simulink model "closed_circuit_simulink"  (R2025b)
settings: Solver=FixedStepDiscrete  StartTime=0.0  StopTime=5  FixedStep=0.01  RelTol=1e-3
values from neighbouring files (symbols this model uses):
  PSD_fresh = PSD_fresh / sum(PSD_fresh)    [Initialisation_simulink.m]    (also in closed_circuit_mill_cyclone.m = data.PSD_fresh_percent(:)' / sum(data.PSD_fresh_percent); closed_circuit_with_pulp.m = PSD_fresh/sum(PSD_fresh))
settings Model: Creator=fabri  LastModifiedBy=fabri
settings DebuggingCC: AlgebraicLoopMsg=none

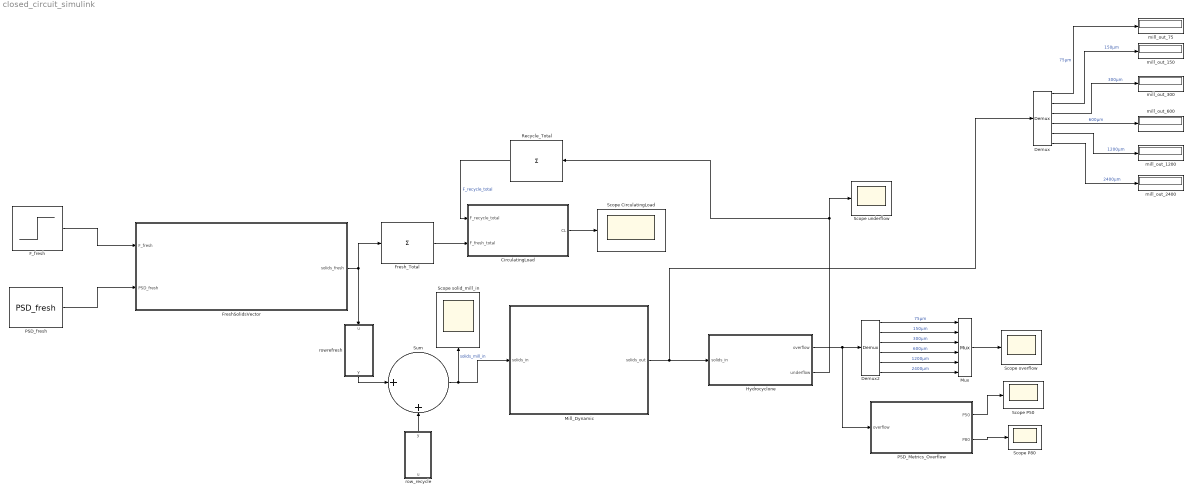
== system closed_circuit_simulink ==
  CirculatingLoad : MATLAB Function  TreatAsAtomicUnit=on
  Demux : Demux  Outputs=6
  Demux2 : Demux  Outputs=6
  F_fresh : Step  Time=2  Before=100  After=120  SampleTime=0
  FreshSolidsVector : MATLAB Function  TreatAsAtomicUnit=on
  Fresh_Total : Sum  Inputs=+
  Hydrocyclone : Subsystem
  Mill_Dynamic : Subsystem
  Mux : Mux  Inputs=6
  PSD_Metrics_Overflow : MATLAB Function  TreatAsAtomicUnit=on
  PSD_fresh : Constant  Value=PSD_fresh
  Recycle_Total : Sum  Inputs=+
  Scope CirculatingLoad : Scope
      settings: ActiveDisplayYMinimum=-0.12499989982802118  ActiveDisplayYMaximum=1.1249990984521909  DataLoggingVariableName=ScopeData3
  Scope P50 : Scope
      settings: ActiveDisplayYMinimum=129.16776995658694  ActiveDisplayYMaximum=136.03382464797281  YLabel=Flow rate (t/h)  DataLoggingVariableName=ScopeData4
  Scope P80 : Scope
      settings: ActiveDisplayYMinimum=262.78762207985039  ActiveDisplayYMaximum=284.16808065274466  YLabel=Flow rate (t/h)  DataLoggingVariableName=ScopeData5
  Scope overflow : Scope
      settings: ActiveDisplayYMinimum=-371.98238867119983  ActiveDisplayYMaximum=1586.5773709597061  YLabel=Flow rate (t/h)
  Scope solid_mill_in : Scope
      settings: ActiveDisplayYMinimum=3.0098879063285189  ActiveDisplayYMaximum=36.512278921953538
  Scope underflow : Scope
      settings: ActiveDisplayYMinimum=-0.69801762722274052  ActiveDisplayYMaximum=1.5006822165423852  DataLoggingVariableName=ScopeData2
  Sum : Sum  Inputs=|++
  mill_out_{75,150,300,600,1200,2400} (6 alike) : Display
  row_recycle : MATLAB Function  TreatAsAtomicUnit=on
  rowrefresh : MATLAB Function  TreatAsAtomicUnit=on
  wires:
  F_fresh/1 -> FreshSolidsVector/1(F_fresh)
  PSD_fresh/1 -> FreshSolidsVector/2(PSD_fresh)
  FreshSolidsVector/1(solids_fresh) -> rowrefresh/1(u), Fresh_Total/1
  Sum/1 -> Mill_Dynamic/1(solids_in), Scope solid_mill_in/1  "solids_mill_in"
  Demux/6 -> mill_out_2400/1  "2400µm"
  Demux/4 -> mill_out_600/1  "600µm"
  Demux/3 -> mill_out_300/1  "300µm"
  Demux/2 -> mill_out_150/1  "150µm"
  Demux/1 -> mill_out_75/1  "75µm"
  Mill_Dynamic/1(solids_out) -> Demux/1, Hydrocyclone/1(solids_in)
  Demux/5 -> mill_out_1200/1  "1200µm"
  Hydrocyclone/2(underflow) -> Scope underflow/1, Recycle_Total/1
  row_recycle/1(y) -> Sum/2
  rowrefresh/1(y) -> Sum/1
  Hydrocyclone/1(overflow) -> Demux2/1, PSD_Metrics_Overflow/1(overflow)
  Demux2/3 -> Mux/3  "300µm"
  Fresh_Total/1 -> CirculatingLoad/2(F_fresh_total)
  Recycle_Total/1 -> CirculatingLoad/1(F_recycle_total)  "F_recycle_total"
  CirculatingLoad/1(CL) -> Scope CirculatingLoad/1
  Mux/1 -> Scope overflow/1
  Demux2/1 -> Mux/1  "75µm"
  Demux2/4 -> Mux/4  "600µm"
  Demux2/2 -> Mux/2  "150µm"
  Demux2/5 -> Mux/5  "1200µm"
  Demux2/6 -> Mux/6  "2400µm"
  PSD_Metrics_Overflow/2(P80) -> Scope P80/1
  PSD_Metrics_Overflow/1(P50) -> Scope P50/1

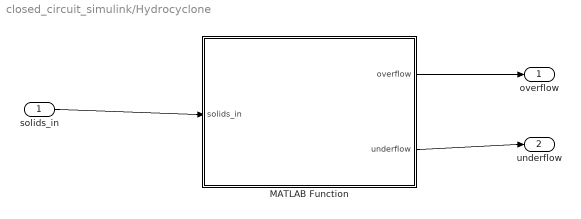
== system closed_circuit_simulink/Hydrocyclone ==
  solids_in : Inport
  MATLAB Function : MATLAB Function  TreatAsAtomicUnit=on
  overflow : Outport
  underflow : Outport  Port=2
  wires:
  solids_in/1 -> MATLAB Function/1(solids_in)
  MATLAB Function/2(underflow) -> underflow/1
  MATLAB Function/1(overflow) -> overflow/1

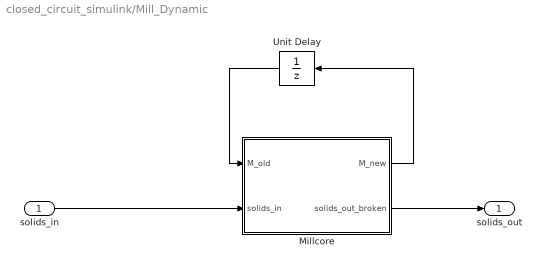
== system closed_circuit_simulink/Mill_Dynamic ==
  solids_in : Inport
  Millcore : MATLAB Function  TreatAsAtomicUnit=on
  Unit Delay : UnitDelay  InitialCondition=[0 0 0 0 0 0]  SampleTime=-1  HasFrameUpgradeWarning=on
  solids_out : Outport
  wires:
  solids_in/1 -> Millcore/2(solids_in)
  Millcore/1(M_new) -> Unit Delay/1
  Millcore/2(solids_out_broken) -> solids_out/1
  Unit Delay/1 -> Millcore/1(M_old)

== matlab function closed_circuit_simulink/Mill_Dynamic/Millcore ==
  data: M_old input; M_new output; solids_in input; solids_out_broken output
function [M_new, solids_out_broken] = MillCore(M_old, solids_in)

% Paramètres
tau = 0.25;
dt  = 0.01;

selection = [0 0.05 0.10 0.20 0.35 0.50];

B = [1   1   0.3 0.1 0   0;
     0   0   0.7 0.3 0.2 0;
     0   0   0   0.6 0.3 0.2;
     0   0   0   0   0.5 0.3;
     0   0   0   0   0   0.5;
     0   0   0   0   0   0];

% Forcer vecteurs ligne
M_old = reshape(M_old, 1, []);
solids_in = reshape(solids_in, 1, []);

% Débit de sortie brut
solids_out_raw = M_old / tau;
F_out = sum(solids_out_raw);

% PSD brute
if F_out > 0
    PSD_raw = solids_out_raw / F_out;
else
    PSD_raw = zeros(size(solids_out_raw));
end

% Application de la cassure
PSD_broken = run_breakage(PSD_raw, selection, B);

% Débit solide broyé en sortie
solids_out_broken = F_out * PSD_broken;

% Bilan dynamique
dMdt = solids_in - solids_out_broken;
M_new = M_old + dt * dMdt;

M_new(M_new < 0) = 0;

end

function PSD_out = run_breakage(PSD_in, selection, B)

n = length(PSD_in);
PSD_out = zeros(1,n);

for j = 1:n
    f = PSD_in(j);
    s = selection(j);

    unbroken = (1-s) * f;
    broken = s * f;

    PSD_out(j) = PSD_out(j) + unbroken;
    PSD_out = PSD_out + broken * B(:,j)';
end

if sum(PSD_out) > 0
    PSD_out = PSD_out / sum(PSD_out);
end

end

== matlab function closed_circuit_simulink/FreshSolidsVector ==
  data: F_fresh input; solids_fresh output; PSD_fresh input
function solids_fresh = FreshSolidsVector(F_fresh, PSD_fresh)

PSD_fresh = reshape(PSD_fresh, 1, []);
solids_fresh = F_fresh .* PSD_fresh;

end

== matlab function closed_circuit_simulink/Hydrocyclone/MATLAB Function ==
  data: solids_in input; overflow output; underflow output
function [overflow, underflow] = CycloneCore(solids_in)

% Paramètre
d50 = 300; % micron (taille de coupure)

size_classes = [75 150 300 600 1200 2400];

% Forcer vecteur ligne
solids_in = reshape(solids_in, 1, []);

F = sum(solids_in);

if F == 0
    overflow = zeros(size(solids_in));
    underflow = zeros(size(solids_in));
    return;
end

PSD = solids_in / F;

% Courbe de partition (simple)
partition = 1 ./ (1 + (size_classes / d50).^2);

% Overflow = fines
PSD_over = PSD .* partition;

% Underflow = gros
PSD_under = PSD .* (1 - partition);

% Normalisation
PSD_over = PSD_over / sum(PSD_over);
PSD_under = PSD_under / sum(PSD_under);

overflow = F * PSD_over;
underflow = F * PSD_under;

end

== matlab function closed_circuit_simulink/rowrefresh ==
  data: u input; y output
function y = RowFresh(u)
y = reshape(u, 1, []);
end

== matlab function closed_circuit_simulink/row_recycle ==
  data: u input; y output
function y = RowRecycle(u)
y = reshape(u, 1, []);
end

== matlab function closed_circuit_simulink/CirculatingLoad ==
  data: F_recycle_total input; CL output; F_fresh_total input
function CL = CirculatingLoad(F_recycle_total, F_fresh_total)

if F_fresh_total <= 0
    CL = 0;
else
    CL = F_recycle_total / F_fresh_total;
end

== matlab function closed_circuit_simulink/PSD_Metrics_Overflow ==
  data: overflow input; P50 output; P80 output
function [P50, P80] = PSD_Metrics_Overflow(overflow)

size_classes = [75 150 300 600 1200 2400];

overflow = reshape(overflow, 1, []);
F = sum(overflow);

if F <= 0
    P50 = NaN;
    P80 = NaN;
    return;
end

PSD = overflow / F;
cumPSD = cumsum(PSD);

P50 = interp_metric(size_classes, cumPSD, 0.50);
P80 = interp_metric(size_classes, cumPSD, 0.80);

end

function D = interp_metric(size_classes, cumulative_curve, target)

if max(cumulative_curve) < target || min(cumulative_curve) > target
    D = NaN;
else
    D = interp1(cumulative_curve, size_classes, target, 'linear');
end

end
